simulink model "chap2_7"  (Simulink 3.00)
settings: Solver=ode45  StartTime=0.0  StopTime=3  RelTol=1e-3
settings Model: LastModifiedBy=liu

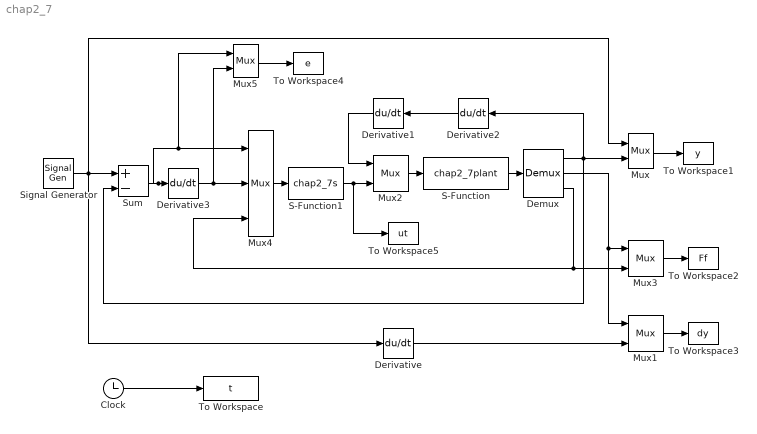
== system chap2_7 ==
  Clock : Clock
      settings: DisplayTime=off  Decimation=10
  Demux : Demux  Outputs=3
  Derivative : Derivative
  Derivative1 : Derivative  Orientation=left
  Derivative2 : Derivative  Orientation=left
  Derivative3 : Derivative
  Mux{,1..3,5} (5 alike) : Mux  Inputs=2
      settings: DisplayOption=none
  Mux4 : Mux  Inputs=3
      settings: DisplayOption=none
  S-Function : S-Function  FunctionName=chap2_7plant  PortCounts=[]  SFunctionModules=''
  S-Function1 : S-Function  FunctionName=chap2_7s  PortCounts=[]  SFunctionModules=''
  Signal Generator : SignalGenerator  WaveForm=sine  Amplitude=0.1  Frequency=1  Units=Hertz
  Sum : Sum  Inputs=+-  SaturateOnIntegerOverflow=on
  To Workspace : ToWorkspace  VariableName=t  SampleTime=-1  SaveFormat=Matrix
  To Workspace1 : ToWorkspace  VariableName=y  SampleTime=-1  SaveFormat=Matrix
  To Workspace2 : ToWorkspace  VariableName=Ff  SampleTime=-1  SaveFormat=Matrix
  To Workspace3 : ToWorkspace  VariableName=dy  SampleTime=-1  SaveFormat=Matrix
  To Workspace4 : ToWorkspace  VariableName=e  SampleTime=-1  SaveFormat=Matrix
  To Workspace5 : ToWorkspace  VariableName=ut  SampleTime=-1  SaveFormat=Matrix
  wires:
  Signal Generator/1 -> Sum/1, Mux/1, Derivative/1
  S-Function/1 -> Demux/1
  Mux2/1 -> S-Function/1
  Derivative1/1 -> Mux2/1
  Derivative2/1 -> Derivative1/1
  Mux4/1 -> S-Function1/1
  Sum/1 -> Derivative3/1, Mux4/1, Mux5/1
  Mux5/1 -> To Workspace4/1
  Derivative3/1 -> Mux4/2, Mux5/2
  S-Function1/1 -> Mux2/2, To Workspace5/1
  Demux/3 -> Mux3/2, Mux4/3
  Demux/1 -> Mux/2, Sum/2, Derivative2/1
  Demux/2 -> Mux1/1, Mux3/1
  Mux3/1 -> To Workspace2/1
  Mux1/1 -> To Workspace3/1
  Derivative/1 -> Mux1/2
  Mux/1 -> To Workspace1/1
  Clock/1 -> To Workspace/1
